simulink model "modos_deslizantes00"  (R2025b)
settings: Solver=VariableStepAuto  StartTime=0.0  StopTime=50  RelTol=1e-3
settings Model: Creator=Lenovo  LastModifiedBy=Lenovo

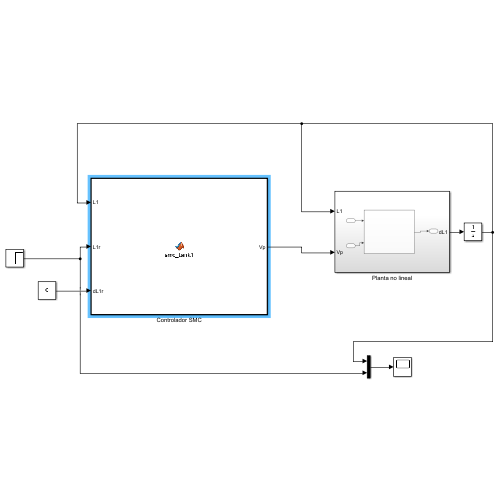
[thumbnail: Simulink's stored preview of the top-level diagram]
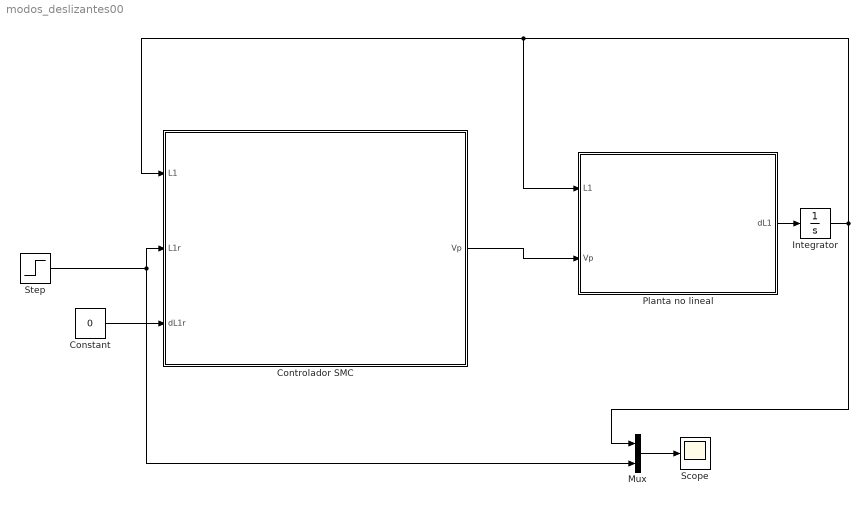
== system modos_deslizantes00 ==
  Constant : Constant  Value=0
  Controlador SMC : MATLAB Function  TreatAsAtomicUnit=on
  Integrator : Integrator
  Mux : Mux  Inputs=2
  Planta no lineal : Subsystem
  Scope : Scope
      settings: ActiveDisplayYMinimum=-0.12499999999999997  ActiveDisplayYMaximum=1.125
  Step : Step  Before=1  SampleTime=0
  wires:
  Planta no lineal/1(dL1) -> Integrator/1
  Integrator/1 -> Planta no lineal/1(L1), Controlador SMC/1(L1), Mux/1
  Controlador SMC/1(Vp) -> Planta no lineal/2(Vp)
  Step/1 -> Mux/2, Controlador SMC/2(L1r)
  Mux/1 -> Scope/1
  Constant/1 -> Controlador SMC/3(dL1r)

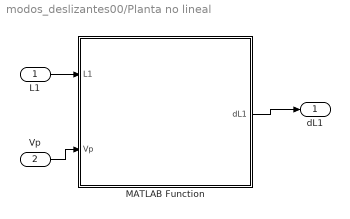
== system modos_deslizantes00/Planta no lineal ==
  L1 : Inport
  Vp : Inport  Port=2
  MATLAB Function : MATLAB Function  TreatAsAtomicUnit=on
  dL1 : Outport
  wires:
  MATLAB Function/1(dL1) -> dL1/1
  L1/1 -> MATLAB Function/1(L1)
  Vp/1 -> MATLAB Function/2(Vp)

== matlab function modos_deslizantes00/Controlador SMC ==
  data: L1 input; Vp output; L1r input; dL1r input
function Vp = smc_tank1(L1, L1r, dL1r)
  % parámetros físicos
  At1 = 15.5179; Ao1 = 0.3167; g = 980; Kp = 3.3;
  b  = Kp/At1; a1 = Ao1*sqrt(2*g)/At1;

  % parámetros SMC
  lambda = 0.2;
  k      = 0.2;
  phi    = 0.05;
  eps    = phi/3;          % para tanh

  % protecciones mínimas
  L1 = max(L1,0);

  e = L1 - L1r;

  % suavizado con tanh (menos abrupto que sat)
  sat_e = tanh(e/eps);

  % ley SMC (pura)
  Vp = ( a1*sqrt(L1) + dL1r - lambda*e - k*sat_e ) / b;
end

== matlab function modos_deslizantes00/Planta no lineal/MATLAB Function ==
  data: dL1 output; L1 input; Vp input
function dL1 = tank1_model(L1, Vp)
% Modelo del tanque 1 (para usar dentro de Simulink MATLAB Function)
% dL1 = b*Vp - a1*sqrt(L1)
% Incluye comprobaciones básicas

% ----- Parámetros físicos (misma unidad: cm, cm^2, cm^3/s) -----
At1 = 15.5179;   % cm^2
Ao1 = 0.3167;    % cm^2
g   = 980;       % cm/s^2
Kp  = 3.3;       % cm^3/(s·V)

% ----- Cálculo de coeficientes -----
b  = Kp / At1;
a1 = Ao1 * sqrt(2*g) / At1;

% ----- Protección numérica -----
L1 = max(L1, 0);        % no negativos
L1 = min(L1, 1e4);      % tope razonable para simulación (evita overflow)

% ----- Dinámica -----
dL1 = b*Vp - a1*sqrt(L1);

end
